simulink model "Vorlage_Course_A_Basis_V01_2021b"  (R2021b)
settings: Solver=FixedStepAuto  StartTime=0.0  StopTime=inf  FixedStep=1e-3  RelTol=1e-3
libraries: simulink x9, instrumentseriallib x3, eeGeneralControl x1
settings Model: Creator=hrebholz  LastModifiedBy=Julian
settings DebuggingCC: ParameterPrecisionLossMsg=none  UnconnectedInputMsg=none  UnconnectedOutputMsg=none  UnconnectedLineMsg=none
settings ModelReferenceCC: EnableRefExpFcnMdlSchedulingChecks=off
settings RTWCC: DLArmComputeVersion=20.02.1

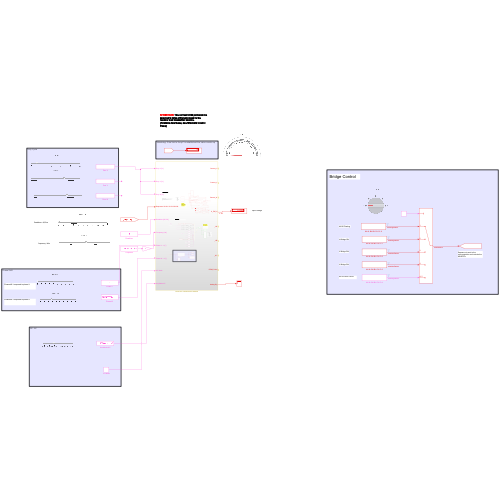
[thumbnail: Simulink's stored preview of the top-level diagram]
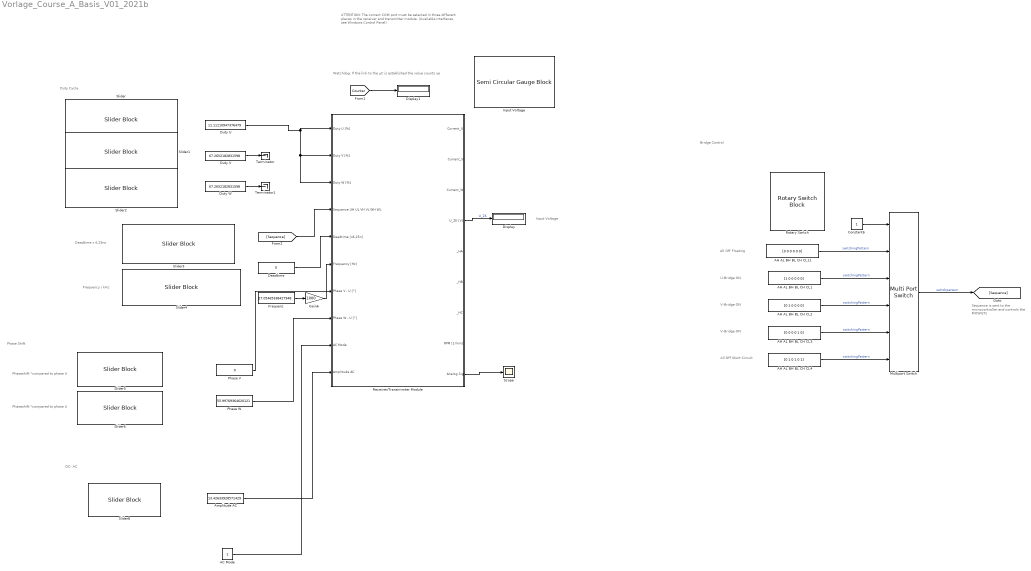
== system Vorlage_Course_A_Basis_V01_2021b ==
  note: Sequence is sent to the microcontroller and controls the MOSFETs
  note: Duty Cycle
  note: Phase Shift
  note: All Off Floating
  note: Watchdog: If the link to the µC is established the value counts up
  note: ATTENTION: The correct COM port must be selected in three different places in the receiver and transmitter module.
      | (Available interfaces, see Windows Control Panel)
  note: Deadtime x 6,25ns
  note: Frequency / kHz
  note: Phaseshift °compared to phase U
  note: Phaseshift °compared to phase U
  note: U-Bridge ON
  note: V-Bridge ON
  note: V-Bridge ON
  note: All Off Short Circuit
  note: Bridge Control
  note: Input Voltage
  note: DC- AC
  AC Mode : Constant
  AH AL BH BL CH CL1 : Constant  Value=[1 0 0 0 0 0]  SampleTime=-1
  AH AL BH BL CH CL11 : Constant  Value=[0 0 0 0 0 0]  SampleTime=-1
  AH AL BH BL CH CL2 : Constant  Value=[0 1 0 0 0 0]  SampleTime=-1
  AH AL BH BL CH CL3 : Constant  Value=[0 0 0 0 1 0]  SampleTime=-1
  AH AL BH BL CH CL4 : Constant  Value=[0 1 0 1 0 1]
  Amplitude AC : Constant  Value=13.42633928571429
  Constant6 : Constant  OutDataTypeStr=uint8
  Deadtime : Constant  Value=0  OutDataTypeStr=uint16
  Display : Display
  Display1 : Display
  Duty U : Constant  Value=11.11110947376479
  Duty V : Constant  Value=67.2652182831598
  Duty W : Constant  Value=67.2652182831598
  Frequenz : Constant  Value=27.05465338427948  OutDataTypeStr=uint16
  Gain6 : Gain  Gain=1000
  Input Voltage : SemiCircularGaugeBlock  ScaleMax=25
  Multiport Switch : MultiPortSwitch  Inputs=5  DiagnosticForDefault=None
  Phase V : Constant  Value=0  OutDataTypeStr=uint16
  Phase W : Constant  Value=55.99769364620121  OutDataTypeStr=uint16
  Receiver/Transimmter Module : Subsystem
  Rotary Switch : RotarySwitchBlock
      settings: Values={{'1', '2', '3', '4', '5'}, [1 2 3 4 5]}
  Scope : Scope
  Slider : SliderBlock  TickInterval=20
  Slider1 : SliderBlock  TickInterval=20
  Slider2 : SliderBlock  TickInterval=20
  Slider3 : SliderBlock  ScaleMax=500  TickInterval=50
  Slider4 : SliderBlock  ScaleMin=1  ScaleMax=50  TickInterval=10
  Slider5 : SliderBlock  ScaleMax=180  TickInterval=20
  Slider6 : SliderBlock  ScaleMax=180  TickInterval=20
  Slider8 : SliderBlock  ScaleMax=36
  Terminator : Terminator
  Terminator1 : Terminator
  wires:
  AH AL BH BL CH CL1/1 -> Multiport Switch/3  "switchingPattern"
  AH AL BH BL CH CL11/1 -> Multiport Switch/2  "switchingPattern"
  AH AL BH BL CH CL2/1 -> Multiport Switch/4  "switchingPattern"
  Multiport Switch/1 -> [Sequence]  "switchpattern"
  AH AL BH BL CH CL3/1 -> Multiport Switch/5  "switchingPattern"
  Constant6/1 -> Multiport Switch/1
  AH AL BH BL CH CL4/1 -> Multiport Switch/6  "switchingPattern"
  [Sequence] -> Receiver/Transimmter Module/4(Sequence UH UL VH VL WH WL)
  [Counter] -> Display1/1
  Duty U/1 -> Receiver/Transimmter Module/3(Duty W [%]), Receiver/Transimmter Module/2(Duty V [%]), Receiver/Transimmter Module/1(Duty U [%])
  Deadtime/1 -> Receiver/Transimmter Module/5(Deadtime [x6,25n])
  Frequenz/1 -> Gain6/1
  Gain6/1 -> Receiver/Transimmter Module/6(Frequency [Hz])
  Phase V/1 -> Receiver/Transimmter Module/7(Phase V - U [°])
  Phase W/1 -> Receiver/Transimmter Module/8(Phase W - U [°])
  Duty V/1 -> Terminator/1
  Duty W/1 -> Terminator1/1
  Receiver/Transimmter Module/4(U_ZK [V]) -> Display/1  "U_ZK"
  Receiver/Transimmter Module/9(Analog Sig) -> Scope/1
  Amplitude AC/1 -> Receiver/Transimmter Module/10(Amplitude AC)
  AC Mode/1 -> Receiver/Transimmter Module/9(AC Mode)

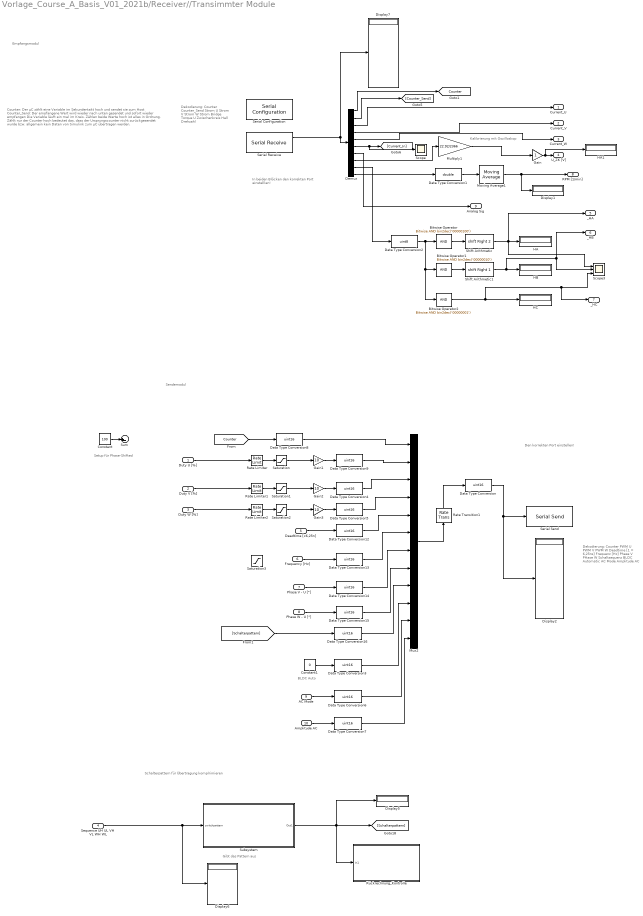
== system Vorlage_Course_A_Basis_V01_2021b/Receiver//Transimmter Module ==
  note: BLDC Auto
  note: Setup für Phase-Shifted
  note: Counter:
      | Der µC zählt eine Variable im Sekundentakt hoch und sendet sie zum Host
      | Counter_Send:
      | Der empfangene Wert wird wieder nach unten gesendet und sofort wieder empfangen
      | Die Variable läuft ein mal im Kreis.
      | Zählen beide Werte hoch ist alles in Ordnung.
      | Zählt nur der Counter hoch bedeutet das, dass der Ursprungscounter nicht zurückgesendet wurde bzw. allgemein kein Daten von Simulink zum µC übertragen werden.
  note: Dekodierung:
      | Counter
      | Counter_Send
      | Strom U
      | Strom V
      | Strom W
      | Strom Bridge
      | Torque
      | U Zwischenkreis
      | Hall
      | Drehzahl
  note: Kalibrierung mit Oszilloskop
  note: Dekodierung:
      | Counter
      | PWM U
      | PWM V
      | PWM W
      | Deadtime [1 = 6,25ns]
      | Frequenz [Hz]
      | Phase V
      | PHase W
      | Schaltsequenz
      | BLDC Automatic
      | AC Mode
      | Amplitude AC
  note: Den korrekten Port einstellen!
  note: Sendemodul
  note: Empfangsmodul
  note: In beiden Blöcken den korrekten Port einstelllen!
  note: Schalterpattern für Übertragung komplrimieren
  note: Gibt das Pattern aus
  Duty U [%] : Inport
  Duty V [%] : Inport  Port=2
  Duty W [%] : Inport  Port=3
  Sequence UH UL VH VL WH WL : Inport  Port=4
  Deadtime [x6,25n] : Inport  Port=5
  Frequency [Hz] : Inport  Port=6
  Phase V - U [°] : Inport  Port=7
  Phase W - U [°] : Inport  Port=8
  AC Mode : Inport  Port=9
  Amplitude AC : Inport  Port=10
  Bitwise Operator : simulink/Logic and Bit Operations/Bitwise Operator  logicop=AND  UseBitMask=on  BitMask=bin2dec('00000100')  BitMaskRealWorld=Stored Integer
  Bitwise Operator1 : simulink/Logic and Bit Operations/Bitwise Operator  logicop=AND  UseBitMask=on  BitMask=bin2dec('00000010')  BitMaskRealWorld=Stored Integer
  Bitwise Operator2 : simulink/Logic and Bit Operations/Bitwise Operator  logicop=AND  UseBitMask=on  BitMask=bin2dec('00000001')  BitMaskRealWorld=Stored Integer
  Constant : Constant  Value=100
  Constant1 : Constant  Value=0
  Data Type Conversion{,3..9,12..16} (13 alike) : DataTypeConversion  OutDataTypeStr=uint16
  Data Type Conversion1 : DataTypeConversion  OutDataTypeStr=double
  Data Type Conversion2 : DataTypeConversion  OutDataTypeStr=uint8
  Demux : Demux  Outputs=10
  Display{1..2,5..7} (5 alike) : Display
  Gain : Gain
  Gain1 : Gain  Gain=10
  Gain2 : Gain  Gain=10
  Gain3 : Gain  Gain=10
  HA : Display
  HA1 : Display
  HB : Display
  HC : Display
  Moving Average1 : eeGeneralControl/Moving Average  VariantControl=Variant1  LabelModeActiveChoice=Discrete  f=2  x0=0  BufferSize=8192  Ts=-1
      settings: SourceProductBaseCode=PS
  Multiply1 : Gain  Gain=22.92/2366
  Mux2 : Mux  Inputs=12
  Rate Limiter : RateLimiter  RisingSlewLimit=200  FallingSlewLimit=-200
  Rate Limiter1 : RateLimiter  RisingSlewLimit=200  FallingSlewLimit=-200
  Rate Limiter2 : RateLimiter  RisingSlewLimit=200  FallingSlewLimit=-200
  Rate Transition1 : RateTransition  OutPortSampleTime=0.05
  Rückrechnung_Kontrolle : Subsystem
  Saturation : Saturate  UpperLimit=90  LowerLimit=0
  Saturation1 : Saturate  UpperLimit=90  LowerLimit=0
  Saturation2 : Saturate  UpperLimit=90  LowerLimit=0
  Saturation3 : Saturate  UpperLimit=100000  LowerLimit=1000
  Scope : Scope
  Scope3 : Scope  NumInputPorts=3
  Serial Configuration : instrumentseriallib/Serial Configuration  Priority=-200000  Port=COM3  ComPort=COM3  BaudRate=115000  DataBits=8  Parity=even  StopBits=1  ByteOrder=little-endian  FlowControl=none  Timeout=10  SimulateUsing=Interpreted execution  BlockInModel=on
  Serial Receive : instrumentseriallib/Serial Receive  Priority=1  Port=COM3  ComPort=COM3  DataType=uint16  SaveDataType=uint8  ToggleHeader=on  Header=['X']  ToggleTerminator=on  Terminator=Custom terminator  CustomTerminator=['Y']  ToggleDataSize=on  DataSize=[1 10]  EnableBlockingMode=off  ActionDataUnavailable=Output last received value  ActionWhenDataUnavailable=Output last received value  CustomValue=42  SampleTime=0.001  SimulateUsing=Interpreted execution  BlockInModel=on
  Serial Send : instrumentseriallib/Serial Send  Priority=1  Port=COM3  ComPort=COM3  Header=[]  Terminator=<none>  CustomTerminator=[]  EnableBlockingMode=off  SimulateUsing=Interpreted execution  BlockInModel=on
  Shift Arithmetic : ArithShift  BitShiftNumber=2  BitShiftDirection=Right
  Shift Arithmetic1 : ArithShift  BitShiftNumber=1  BitShiftDirection=Right
  Subsystem : Subsystem
  Sum : Sum  Inputs=|+-
  Current_U : Outport
  Current_V : Outport  Port=2
  Current_W : Outport  Port=3
  U_ZK [V] : Outport  Port=4
  _HA : Outport  Port=5
  _HB : Outport  Port=6
  _HC : Outport  Port=7
  " RPM [1/min]" : Outport  Port=8
  Analog Sig : Outport  Port=9
  tag scope: Counter=global
  wires:
  Demux/4 -> Current_V/1
  Data Type Conversion1/1 -> Moving Average1/1
  Serial Receive/1 -> Demux/1, Display7/1
  Demux/3 -> Current_U/1
  Moving Average1/1 -> " RPM [1/min]"/1, Display1/1
  Demux/5 -> Current_W/1
  Demux/6 -> Scope/1, [Current_In]
  Demux/2 -> [Counter_Send]
  Multiply1/1 -> Gain/1
  Demux/10 -> Data Type Conversion1/1
  Bitwise Operator1/1 -> Shift Arithmetic1/1
  Data Type Conversion2/1 -> Bitwise Operator2/1, Bitwise Operator1/1, Bitwise Operator/1
  Bitwise Operator/1 -> Shift Arithmetic/1
  Shift Arithmetic/1 -> _HA/1, Scope3/1, HA/1
  Shift Arithmetic1/1 -> _HB/1, Scope3/2, HB/1
  Bitwise Operator2/1 -> HC/1, _HC/1, Scope3/3
  Demux/8 -> Multiply1/1
  Demux/9 -> Data Type Conversion2/1
  Demux/1 -> [Counter]
  Data Type Conversion15/1 -> Mux2/8
  Data Type Conversion12/1 -> Mux2/5
  Data Type Conversion16/1 -> Mux2/9
  Data Type Conversion13/1 -> Mux2/6
  Data Type Conversion8/1 -> Mux2/1
  Data Type Conversion9/1 -> Mux2/2
  Rate Transition1/1 -> Data Type Conversion/1
  Mux2/1 -> Rate Transition1/1
  Gain1/1 -> Data Type Conversion9/1
  Duty U [%]/1 -> Rate Limiter/1
  Data Type Conversion/1 -> Display2/1, Serial Send/1
  Data Type Conversion14/1 -> Mux2/7
  Data Type Conversion3/1 -> Mux2/10
  [Counter] -> Data Type Conversion8/1
  Gain/1 -> HA1/1, U_ZK [V]/1
  Gain2/1 -> Data Type Conversion4/1
  Data Type Conversion4/1 -> Mux2/3
  Data Type Conversion5/1 -> Mux2/4
  Gain3/1 -> Data Type Conversion5/1
  Duty W [%]/1 -> Rate Limiter2/1
  Subsystem/1(Out1) -> Rückrechnung_Kontrolle/1(In1), [Schalterpattern], Display5/1
  Sequence UH UL VH VL WH WL/1 -> Display6/1, Subsystem/1(switchpattern)
  [Schalterpattern] -> Data Type Conversion16/1
  Rate Limiter/1 -> Saturation/1
  Rate Limiter1/1 -> Saturation1/1
  Rate Limiter2/1 -> Saturation2/1
  Constant/1 -> Sum/1
  Duty V [%]/1 -> Rate Limiter1/1
  Deadtime [x6,25n]/1 -> Data Type Conversion12/1
  Constant1/1 -> Data Type Conversion3/1
  Phase V - U [°]/1 -> Data Type Conversion14/1
  Phase W - U [°]/1 -> Data Type Conversion15/1
  Saturation/1 -> Gain1/1
  Saturation1/1 -> Gain2/1
  Saturation2/1 -> Gain3/1
  Frequency [Hz]/1 -> Data Type Conversion13/1
  Demux/7 -> Analog Sig/1
  AC Mode/1 -> Data Type Conversion6/1
  Amplitude AC/1 -> Data Type Conversion7/1
  Data Type Conversion6/1 -> Mux2/11
  Data Type Conversion7/1 -> Mux2/12

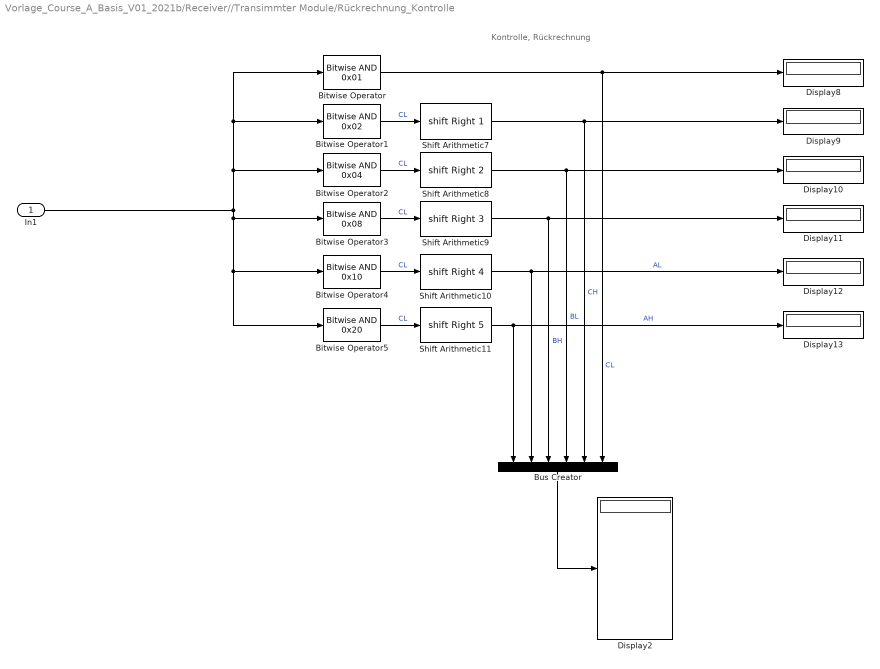
== system Vorlage_Course_A_Basis_V01_2021b/Receiver//Transimmter Module/Rückrechnung_Kontrolle ==
  note: Kontrolle, Rückrechnung
  In1 : Inport
  Bitwise Operator : simulink/Logic and Bit Operations/Bitwise Operator  logicop=AND  UseBitMask=on  BitMask=0x01  BitMaskRealWorld=Stored Integer
  Bitwise Operator1 : simulink/Logic and Bit Operations/Bitwise Operator  logicop=AND  UseBitMask=on  BitMask=0x02  BitMaskRealWorld=Stored Integer
  Bitwise Operator2 : simulink/Logic and Bit Operations/Bitwise Operator  logicop=AND  UseBitMask=on  BitMask=0x04  BitMaskRealWorld=Stored Integer
  Bitwise Operator3 : simulink/Logic and Bit Operations/Bitwise Operator  logicop=AND  UseBitMask=on  BitMask=0x08  BitMaskRealWorld=Stored Integer
  Bitwise Operator4 : simulink/Logic and Bit Operations/Bitwise Operator  logicop=AND  UseBitMask=on  BitMask=0x10  BitMaskRealWorld=Stored Integer
  Bitwise Operator5 : simulink/Logic and Bit Operations/Bitwise Operator  logicop=AND  UseBitMask=on  BitMask=0x20  BitMaskRealWorld=Stored Integer
  Bus Creator : BusCreator  Inputs=6
  Display{2,8..13} (7 alike) : Display
  Shift Arithmetic10 : ArithShift  BitShiftNumber=4  BitShiftDirection=Right
  Shift Arithmetic11 : ArithShift  BitShiftNumber=5  BitShiftDirection=Right
  Shift Arithmetic7 : ArithShift  BitShiftNumber=1  BitShiftDirection=Right
  Shift Arithmetic8 : ArithShift  BitShiftNumber=2  BitShiftDirection=Right
  Shift Arithmetic9 : ArithShift  BitShiftNumber=3  BitShiftDirection=Right
  wires:
  Shift Arithmetic8/1 -> Bus Creator/4, Display10/1  "BL"
  Shift Arithmetic9/1 -> Bus Creator/3, Display11/1  "BH"
  In1/1 -> Bitwise Operator/1, Bitwise Operator1/1, Bitwise Operator2/1, Bitwise Operator5/1, Bitwise Operator4/1, Bitwise Operator3/1
  Bitwise Operator2/1 -> Shift Arithmetic8/1  "CL"
  Shift Arithmetic7/1 -> Bus Creator/5, Display9/1  "CH"
  Shift Arithmetic10/1 -> Display12/1, Bus Creator/2  "AL"
  Bitwise Operator5/1 -> Shift Arithmetic11/1  "CL"
  Shift Arithmetic11/1 -> Display13/1, Bus Creator/1  "AH"
  Bitwise Operator/1 -> Bus Creator/6, Display8/1  "CL"
  Bus Creator/1 -> Display2/1
  Bitwise Operator1/1 -> Shift Arithmetic7/1  "CL"
  Bitwise Operator4/1 -> Shift Arithmetic10/1  "CL"
  Bitwise Operator3/1 -> Shift Arithmetic9/1  "CL"

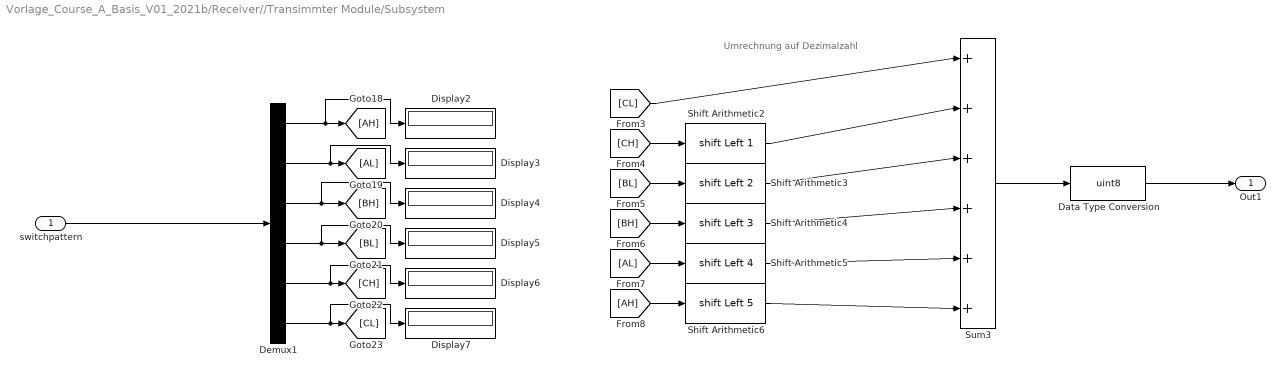
== system Vorlage_Course_A_Basis_V01_2021b/Receiver//Transimmter Module/Subsystem ==
  note: Umrechnung auf Dezimalzahl
  switchpattern : Inport
  Data Type Conversion : DataTypeConversion  OutDataTypeStr=uint8
  Demux1 : Demux  Outputs=6
  Display{2..7} (6 alike) : Display
  Shift Arithmetic2 : ArithShift  BitShiftNumber=1  BitShiftDirection=Left
  Shift Arithmetic3 : ArithShift  BitShiftNumber=2  BitShiftDirection=Left
  Shift Arithmetic4 : ArithShift  BitShiftNumber=3  BitShiftDirection=Left
  Shift Arithmetic5 : ArithShift  BitShiftNumber=4  BitShiftDirection=Left
  Shift Arithmetic6 : ArithShift  BitShiftNumber=5  BitShiftDirection=Left
  Sum3 : Sum  Inputs=|++++++
  Out1 : Outport
  wires:
  [CL] -> Sum3/1
  Demux1/2 -> Display3/1, [AL]
  Demux1/4 -> [BL], Display5/1
  Demux1/5 -> Display6/1, [CH]
  Demux1/3 -> Display4/1, [BH]
  Shift Arithmetic4/1 -> Sum3/4
  Shift Arithmetic2/1 -> Sum3/2
  Demux1/1 -> [AH], Display2/1
  Data Type Conversion/1 -> Out1/1
  [AL] -> Shift Arithmetic5/1
  Demux1/6 -> Display7/1, [CL]
  [CH] -> Shift Arithmetic2/1
  Shift Arithmetic3/1 -> Sum3/3
  Shift Arithmetic6/1 -> Sum3/6
  [BH] -> Shift Arithmetic4/1
  [AH] -> Shift Arithmetic6/1
  Sum3/1 -> Data Type Conversion/1
  Shift Arithmetic5/1 -> Sum3/5
  [BL] -> Shift Arithmetic3/1
  switchpattern/1 -> Demux1/1
